simulink model "examples_of_demux_block"  (R2021a)
settings: Solver=VariableStepAuto  StartTime=0.0  StopTime=1  RelTol=1e-3
settings Model: Creator=YasserNet  LastModifiedBy=YasserNet

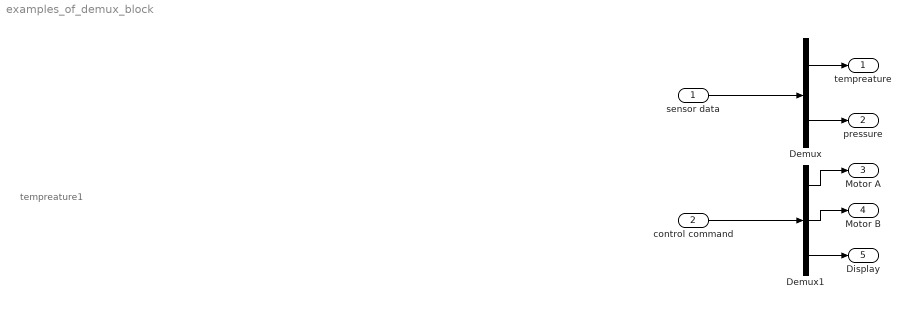
== system examples_of_demux_block ==
  note: tempreature1
  sensor data : Inport
  control command : Inport  Port=2
  Demux : Demux  Outputs=2
  Demux1 : Demux  Outputs=3
  tempreature : Outport
  pressure : Outport  Port=2
  Motor A : Outport  Port=3
  Motor B : Outport  Port=4
  Display : Outport  Port=5
  wires:
  Demux1/3 -> Display/1
  sensor data/1 -> Demux/1
  Demux1/1 -> Motor A/1
  control command/1 -> Demux1/1
  Demux1/2 -> Motor B/1
  Demux/2 -> pressure/1
  Demux/1 -> tempreature/1
